simulink library "dlbsBlockAdd"  (R2025b)
settings: Solver=VariableStepAuto  StartTime=0.0  StopTime=10.0  RelTol=1e-3
libraries: dlbsBlockInsertGradientGF x4, dlbsBlockExtractGradientGF x2, dlbsBlockSumOverMultipleDimensions x2
settings Model: Creator=lt6037  LastModifiedBy=lt6037

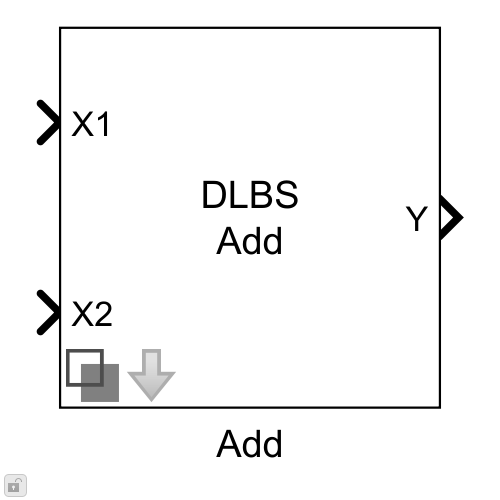
[thumbnail: Simulink's stored preview of the top-level diagram]
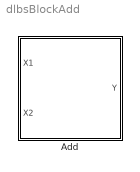
== system dlbsBlockAdd ==
  Add : Subsystem  Variant=on  VariantControlMode=label  LabelModeActiveChoice=no broadcast  mask{broadcast=off, dims1=1, dims2=1}
      mask prompts: broadcast "Broadcast Dimensions"; dims1 "Dimensions to sum over"; dims2 "Dimensions to sum over"
      mask help:
      | Adds two inputs element-wise.
      | This block supports broadcasting, which allows it to add tensors of different sizes together under certain conditions.
      | When broadcasting is enabled, the block can automatically expand certain dimensions of the input tensors to make their sizes compatible for element-wise addition. These dimensions must be of length 1 and must be specified using the 'Dimensions to sum over' parameters for each input.
      mask Help: web("dlbsHelpBlockAdd.html")
      mask TypeOptions dims1: Add Broadcast/dims1
      mask TypeOptions dims2: Add Broadcast/dims2
      mask Display:
      | s = [...
      |     "DLBS",...
      |     "Add"];
      | 
      | 
      | s.append("2");
      | 
      | 
      | if strcmp(get_param(gcbh,"broadcast"),"on")
      |     bc1 = get_param(gcbh,"dims1");
      |     bc2 = get_param(gcbh,"dims2");
      |     s(end+1)="";
      |     s(end+1)=sprintf("X1 Dims: [%s]", bc1);
      |     s(end+1)=sprintf("X2 Dims: [%s]", bc2);
      | end
      | 
      | fprintf(join(s,"\n"));

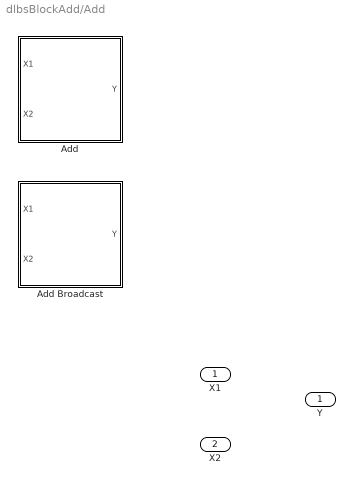
== system dlbsBlockAdd/Add ==
  X1 : Inport
  X2 : Inport  Port=2
  Add : Subsystem  VariantControl=no broadcast
      mask help: Default Mask
  Add Broadcast : Subsystem  VariantControl=broadcast  mask{dims1=dims1, dims2=dims2}
      mask prompts: dims1 "Dimensions to sum over"; dims2 "Dimensions to sum over"
      mask help: Default Mask
      mask TypeOptions dims1: Sum Over Multiple Dimensions x1/dims
      mask TypeOptions dims2: Sum Over Multiple Dimensions x2/dims
  Y : Outport

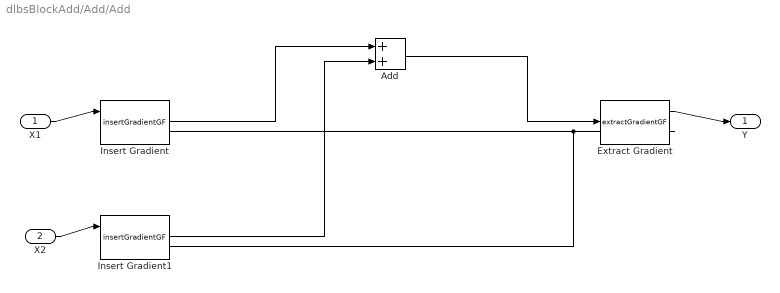
== system dlbsBlockAdd/Add/Add ==
  X1 : Inport
  X2 : Inport  Port=2
  Add : Sum
  Extract Gradient : dlbsBlockExtractGradientGF/extractGradientGF
  Insert Gradient : dlbsBlockInsertGradientGF/insertGradientGF
  Insert Gradient1 : dlbsBlockInsertGradientGF/insertGradientGF
  Y : Outport
  wires:
  Insert Gradient1/1 -> Add/2
  Insert Gradient/1 -> Add/1
  Add/1 -> Extract Gradient/1
  Extract Gradient/2 -> Insert Gradient1/2, Insert Gradient/2
  X1/1 -> Insert Gradient/1
  X2/1 -> Insert Gradient1/1
  Extract Gradient/1 -> Y/1

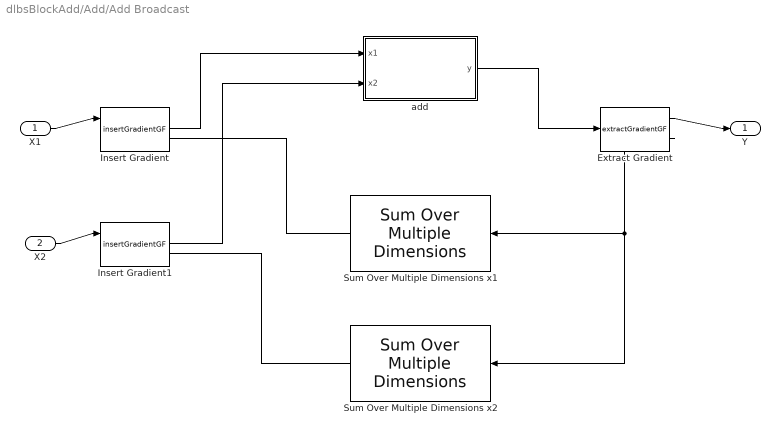
== system dlbsBlockAdd/Add/Add Broadcast ==
  X1 : Inport
  X2 : Inport  Port=2
  Extract Gradient : dlbsBlockExtractGradientGF/extractGradientGF
  Insert Gradient : dlbsBlockInsertGradientGF/insertGradientGF
  Insert Gradient1 : dlbsBlockInsertGradientGF/insertGradientGF
  Sum Over Multiple Dimensions x1 : dlbsBlockSumOverMultipleDimensions/Sum Over Multiple Dimensions  dims=dims1
  Sum Over Multiple Dimensions x2 : dlbsBlockSumOverMultipleDimensions/Sum Over Multiple Dimensions  dims=dims2
  add : MATLAB Function  TreatAsAtomicUnit=on
  Y : Outport
  wires:
  Insert Gradient/1 -> add/1(x1)
  Insert Gradient1/1 -> add/2(x2)
  add/1(y) -> Extract Gradient/1
  Sum Over Multiple Dimensions x1/1 -> Insert Gradient/2
  Sum Over Multiple Dimensions x2/1 -> Insert Gradient1/2
  Extract Gradient/2 -> Sum Over Multiple Dimensions x2/1, Sum Over Multiple Dimensions x1/1
  X1/1 -> Insert Gradient/1
  Extract Gradient/1 -> Y/1
  X2/1 -> Insert Gradient1/1

== matlab function dlbsBlockAdd/Add/Add Broadcast/add ==
  data: y output; x1 input; x2 input
function y   = add_broadcast(x1, x2)

y = x1+x2;

end
